simulink model "arduino"  (R2014a)
settings: Solver=ode3  SolverMode=SingleTasking  StartTime=0.0  StopTime=10.0  RelTol=1e-3
values from neighbouring files (symbols this model uses):
  K_full = lqr(A_full,B_full,[0 0 0 0 0;0 0 0 0 0;0 0 0 0 0;0 0 0 0 0;0 0 0 0 0.5],50)    [LQR_controller.m]
libraries: arduinolib x6
settings Model: SimulationMode=external  ExtModeTrigDuration=2  Creator=Abdelrahman  LastModifiedBy=Abdelrahman
settings OptimizationCC: OptimizeModelRefInitCode=on  LifeSpan=1
settings DebuggingCC: UnderspecifiedInitializationDetection=Classic  SolverPrmCheckMsg=none
settings HardwareCC: ProdBitPerInt=16  ProdBitPerPointer=8  ProdIntDivRoundTo=Zero  ProdEndianess=LittleEndian  ProdWordSize=8  ProdHWDeviceType=Atmel->AVR
settings RTWCC: SystemTargetFile=realtime.tlc  GenerateMakefile=off  TemplateMakefile=realtime.tmf  Description=Run on Target Hardware  RTWVerbose=off  ProcessScript=realtime_make_rtw_hook
settings STFCustomTargetCC: TargetLibSuffix=.a  GenerateSampleERTMain=on  ConcurrentExecutionCompliant=off  GeneratePreprocessorConditionals=Use local settings  ERTCustomFileBanners=on  SupportNonInlinedSFcns=off  SupportVariableSizeSignals=on  MATLABClassNameForMDSCustomization=Simulink.SoftwareTarget.ERTCustomization  GRTInterface=off  SystemTargetFile=realtime.tlc
settings ERTTargetCC: CombineOutputUpdateFcns=off  SupportContinuousTime=on  SupportVariableSizeSignals=on  ExtModeTransport=3  ExtModeMexFile=ext_serial_win32_comm  ExtModeMexArgs=0 1 9600  ERTSrcFileBannerTemplate=realtime_code_template.cgt  ERTHdrFileBannerTemplate=realtime_code_template.cgt  ERTDataSrcFileTemplate=realtime_code_template.cgt  ERTDataHdrFileTemplate=realtime_code_template.cgt  ERTCustomFileTemplate=realtime_file_process.tlc

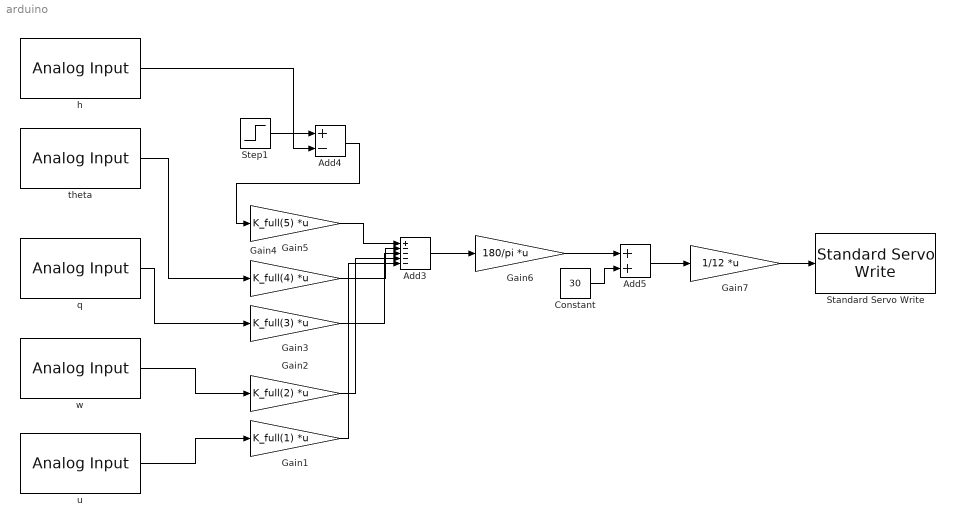
== system arduino ==
  Add3 : Sum  Inputs=+----
  Add4 : Sum  Inputs=+-
  Add5 : Sum
  Constant : Constant  Value=30
  Gain1 : Gain  Gain=K_full(1)  Multiplication=Matrix(K*u)
  Gain2 : Gain  Gain=K_full(2)  Multiplication=Matrix(K*u)
  Gain3 : Gain  Gain=K_full(3)  Multiplication=Matrix(K*u)
  Gain4 : Gain  Gain=K_full(4)  Multiplication=Matrix(K*u)
  Gain5 : Gain  Gain=K_full(5)  Multiplication=Matrix(K*u)
  Gain6 : Gain  Gain=180/pi  Multiplication=Matrix(K*u)
  Gain7 : Gain  Gain=1/12  Multiplication=Matrix(K*u)
  Standard Servo Write : arduinolib/Standard Servo Write  pinNumber=9
  Step1 : Step  After=15  SampleTime=0
  h : arduinolib/Analog Input  pinNumber=0  sampleTime=1
  q : arduinolib/Analog Input  pinNumber=2  sampleTime=1
  theta : arduinolib/Analog Input  pinNumber=1  sampleTime=1
  u : arduinolib/Analog Input  pinNumber=4  sampleTime=1
  w : arduinolib/Analog Input  pinNumber=3  sampleTime=1
  wires:
  theta/1 -> Gain4/1
  q/1 -> Gain3/1
  w/1 -> Gain2/1
  u/1 -> Gain1/1
  Gain5/1 -> Add3/1
  Gain4/1 -> Add3/2
  Gain3/1 -> Add3/3
  Gain2/1 -> Add3/4
  Gain1/1 -> Add3/5
  Step1/1 -> Add4/1
  h/1 -> Add4/2
  Add4/1 -> Gain5/1
  Constant/1 -> Add5/2
  Add5/1 -> Gain7/1
  Gain7/1 -> Standard Servo Write/1
  Add3/1 -> Gain6/1
  Gain6/1 -> Add5/1
